simulink model "PID_example"  (R2012b)
settings: Solver=ode1  StartTime=0.0  StopTime=80  FixedStep=0.01  RelTol=1e-3
StopFcn:
  | plot(time,[Input simout simout1 simout2]);legend('Input','No Windup','Incremental','Back Compute');grid;
  | title('Comparison of PID with and without Anti-Windup')
  | xlabel('Time (sec)');ylabel('Magnitude')
  | shg
undefined symbols (not defined in the file): DiscIntNeverNeededParam, sigbuilder_block
libraries: simulink x3
settings Model: Creator=JYOGANAN  LastModifiedBy=JYOGANAN

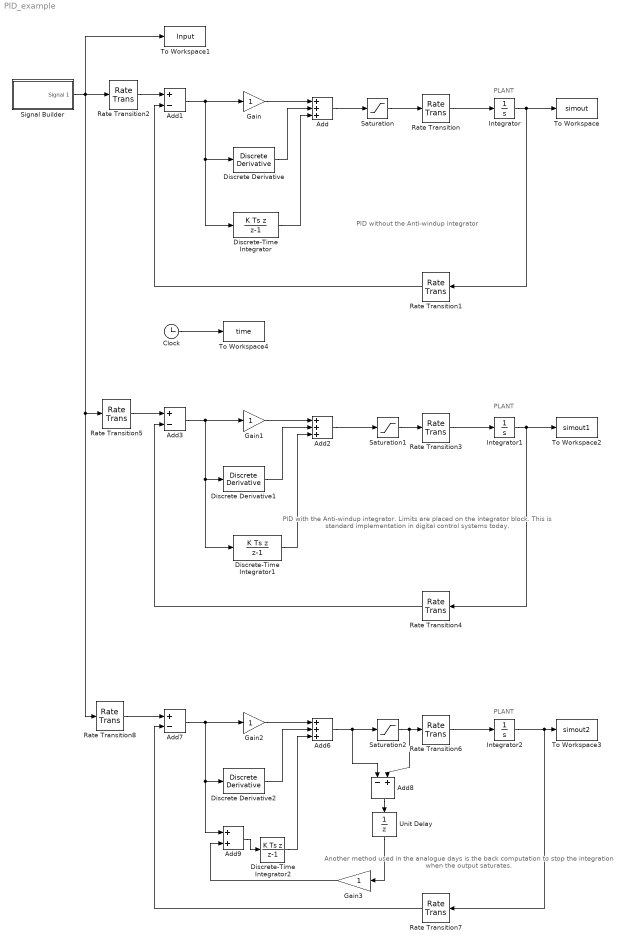
== system PID_example ==
  note: PLANT
  note: PID without the Anti-windup integrator
  note: PID with the Anti-windup integrator.
      | Limits are placed on the integrator block.
      | This is standard implementation in digital
      | control systems today.
  note: Another method used in the analogue days is
      | the back computation to stop the integration
      | when the output saturates.
  note: PLANT
  note: PLANT
  Add : Sum  Inputs=+++
  Add1 : Sum  Inputs=+-
  Add2 : Sum  Inputs=+++
  Add3 : Sum  Inputs=+-
  Add6 : Sum  Inputs=+++
  Add7 : Sum  Inputs=+-
  Add8 : Sum  Inputs=-+
  Add9 : Sum
  Clock : Clock
  Discrete Derivative : simulink/Discrete/Discrete Derivative  gainval=1.0  ICPrevScaledInput=0.0  InputProcessing=Inherited  OutMin=[]  OutMax=[]  OutDataType=fixdt(1, 16)  OutScaling=2^-10  DoSatur=off
  Discrete Derivative1 : simulink/Discrete/Discrete Derivative  gainval=1.0  ICPrevScaledInput=0.0  InputProcessing=Inherited  OutMin=[]  OutMax=[]  OutDataType=fixdt(1, 16)  OutScaling=2^-10  DoSatur=off
  Discrete Derivative2 : simulink/Discrete/Discrete Derivative  gainval=1.0  ICPrevScaledInput=0.0  InputProcessing=Inherited  OutMin=[]  OutMax=[]  OutDataType=fixdt(1, 16)  OutScaling=2^-10  DoSatur=off
  Discrete-Time Integrator : DiscreteIntegrator  IntegratorMethod=Integration: Backward Euler  SampleTime=0.01  UpperSaturationLimit=0.002  LowerSaturationLimit=-0.002  ICPrevOutput=DiscIntNeverNeededParam  ICPrevScaledInput=DiscIntNeverNeededParam
  Discrete-Time Integrator1 : DiscreteIntegrator  IntegratorMethod=Integration: Backward Euler  SampleTime=0.01  LimitOutput=on  UpperSaturationLimit=0.02  LowerSaturationLimit=-0.02  ICPrevOutput=DiscIntNeverNeededParam  ICPrevScaledInput=DiscIntNeverNeededParam
      settings: AttributesFormatString=LL = %<LowerSaturationLimit>\nUL = %<UpperSaturationLimit>
  Discrete-Time Integrator2 : DiscreteIntegrator  IntegratorMethod=Integration: Backward Euler  SampleTime=0.01  UpperSaturationLimit=0.02  LowerSaturationLimit=-0.02  ICPrevOutput=DiscIntNeverNeededParam  ICPrevScaledInput=DiscIntNeverNeededParam
  Gain{,1..3} (4 alike) : Gain
  Integrator : Integrator
  Integrator1 : Integrator
  Integrator2 : Integrator
  Rate Transition : RateTransition
  Rate Transition{1..2,4..5,7..8} (6 alike) : RateTransition  OutPortSampleTime=0.01
  Rate Transition3 : RateTransition
  Rate Transition6 : RateTransition
  Saturation : Saturate  UpperLimit=0.1  LowerLimit=-0.1
  Saturation1 : Saturate  UpperLimit=0.1  LowerLimit=-0.1
  Saturation2 : Saturate  UpperLimit=0.1  LowerLimit=-0.1
  Signal Builder : Subsystem  Tag=STV Subsys  LoadFcn=sigbuilder_block('load');  StartFcn=sigbuilder_block('start');  StopFcn=sigbuilder_block('stop');  ClipboardFcn=sigbuilder_block('clipboard');  mask(Sigbuilder block){}
      mask help: Simulink:masks:SigbuilderBlock_MD
      mask init:
      | if ~strcmp(get_param(bdroot(gcbh),'SimulationStatus'),'stopped') tuvar = sigbuilder_block('maskInit'); end
      settings: CopyFcn=sigbuilder_block('copy');  DeleteFcn=sigbuilder_block('delete');  ModelCloseFcn=sigbuilder_block('modelClose');  PreSaveFcn=sigbuilder_block('preSave');  PauseFcn=sigbuilder_block('pause');  ContinueFcn=sigbuilder_block('continue');  NameChangeFcn=sigbuilder_block('namechange');  OpenFcn=sigbuilder_block('open',[406.5 147 550.5 399.75 ]);  CloseFcn=sigbuilder_block('close');
      mask Display: plot(0, 0, 100, 100,[2, 2, 32, 32, 2], [68, 8, 8, 68, 68],[32, 2], [38, 38], [32, 19, 2],[53, 60, 44], [32, 17, 17, 2],[16, 16, 31, 31]);txt = getActiveGroup(gcbh);text(2, 100, txt,'verticalAlignment', 'top');
  To Workspace : ToWorkspace  VariableName=simout  SampleTime=-1
  To Workspace1 : ToWorkspace  VariableName=Input  SampleTime=-1
  To Workspace2 : ToWorkspace  VariableName=simout1  SampleTime=-1
  To Workspace3 : ToWorkspace  VariableName=simout2  SampleTime=-1
  To Workspace4 : ToWorkspace  VariableName=time  SampleTime=-1
  Unit Delay : UnitDelay  SampleTime=-1
  wires:
  Rate Transition/1 -> Integrator/1
  Add/1 -> Saturation/1
  Saturation/1 -> Rate Transition/1
  Gain/1 -> Add/1
  Discrete Derivative/1 -> Add/2
  Discrete-Time Integrator/1 -> Add/3
  Rate Transition1/1 -> Add1/2
  Add1/1 -> Discrete Derivative/1, Discrete-Time Integrator/1, Gain/1
  Integrator/1 -> To Workspace/1, Rate Transition1/1
  Rate Transition2/1 -> Add1/1
  Rate Transition3/1 -> Integrator1/1
  Gain1/1 -> Add2/1
  Discrete-Time Integrator1/1 -> Add2/3
  Rate Transition4/1 -> Add3/2
  Integrator1/1 -> To Workspace2/1, Rate Transition4/1
  Rate Transition5/1 -> Add3/1
  Discrete Derivative1/1 -> Add2/2
  Saturation1/1 -> Rate Transition3/1
  Add2/1 -> Saturation1/1
  Add3/1 -> Discrete-Time Integrator1/1, Discrete Derivative1/1, Gain1/1
  Signal Builder/1(Signal 1) -> To Workspace1/1, Rate Transition2/1, Rate Transition5/1, Rate Transition8/1
  Rate Transition6/1 -> Integrator2/1
  Gain2/1 -> Add6/1
  Discrete-Time Integrator2/1 -> Add6/3
  Rate Transition7/1 -> Add7/2
  Integrator2/1 -> To Workspace3/1, Rate Transition7/1
  Rate Transition8/1 -> Add7/1
  Discrete Derivative2/1 -> Add6/2
  Saturation2/1 -> Add8/2, Rate Transition6/1
  Add6/1 -> Add8/1, Saturation2/1
  Add9/1 -> Discrete-Time Integrator2/1
  Add7/1 -> Add9/1, Discrete Derivative2/1, Gain2/1
  Add8/1 -> Unit Delay/1
  Clock/1 -> To Workspace4/1
  Gain3/1 -> Add9/2
  Unit Delay/1 -> Gain3/1

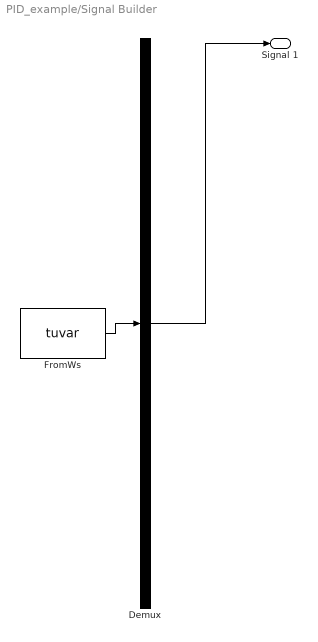
== system PID_example/Signal Builder ==
  Demux : Demux  Tag=STV Demux  Outputs=1
  FromWs : FromWorkspace  Tag=STV FromWs  VariableName=tuvar  SampleTime=0
      SigBuilderData=|
      | common.afterFinalStr = 'Extrapolate'
      | common.sampleTime = 0
      | dataSet.timeRange = [0 80]
      | dataSet.name = 'Group 1'
      | sbobj.Groups.Name = 'Group 1'
      | sbobj.Groups.Signals.Name = 'Signal 1'
      | sbobj.Groups.Signals.XData = [0 26.2 26.2 60 60 72 72 80]
      | sbobj.Groups.Signals.YData = [1 1 -1 -1 1 1 0 0]
      | sbobj.Groups.TimeRange = [0 80]
  Signal 1 : Outport  Tag=STV Outport
  wires:
  Demux/1 -> Signal 1/1
  FromWs/1 -> Demux/1
